simulink model "InductionCookerStateFlow_HarnessInductionCookerS11"  (R2023a)
settings: Solver=FixedStepDiscrete  StartTime=0.0  StopTime=2000  FixedStep=0.1  RelTol=1e-3  EnableMultiTasking=on
settings Model: Creator=antonio  LastModifiedBy=anton
settings SolverCC: AlgebraicLoopSolver=TrustRegion  AutoInsertRateTranBlk=on
settings DataIOCC: LimitDataPoints=on
settings OptimizationCC: LifeSpan=inf
settings DebuggingCC: UnconnectedInputMsg=warning  UnconnectedOutputMsg=warning  UnconnectedLineMsg=warning  AllowSymbolicDim=off  SFUnexpectedBacktrackingDiag=warning  SFNoUnconditionalDefaultTransitionDiag=warning  SFExecutionAtInitializationDiag=none  ArithmeticOperatorsInVariantConditions=warning
settings ModelReferenceCC: EnableRefExpFcnMdlSchedulingChecks=on
settings SFSimCC: SimUseLocalCustomCode=off  CustomCodeUndefinedFunction=UseInterfaceOnly
settings RTWCC: RTWUseLocalCustomCode=off  DLArmComputeVersion=19.05
settings CodeAppCC: StateflowObjectComments=on
settings GRTTargetCC: TargetLangStandard=C89/C90 (ANSI)
settings ConfigComp: CovEnable=on  RecordCoverage=on  CovMetricSettings=dw  CovSaveCumulativeToWorkspaceVar=on  CovSaveSingleToWorkspaceVar=on  CovModelRefEnable=on

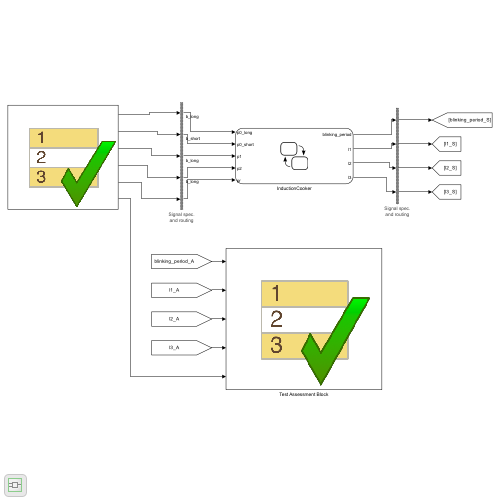
[thumbnail: Simulink's stored preview of the top-level diagram]
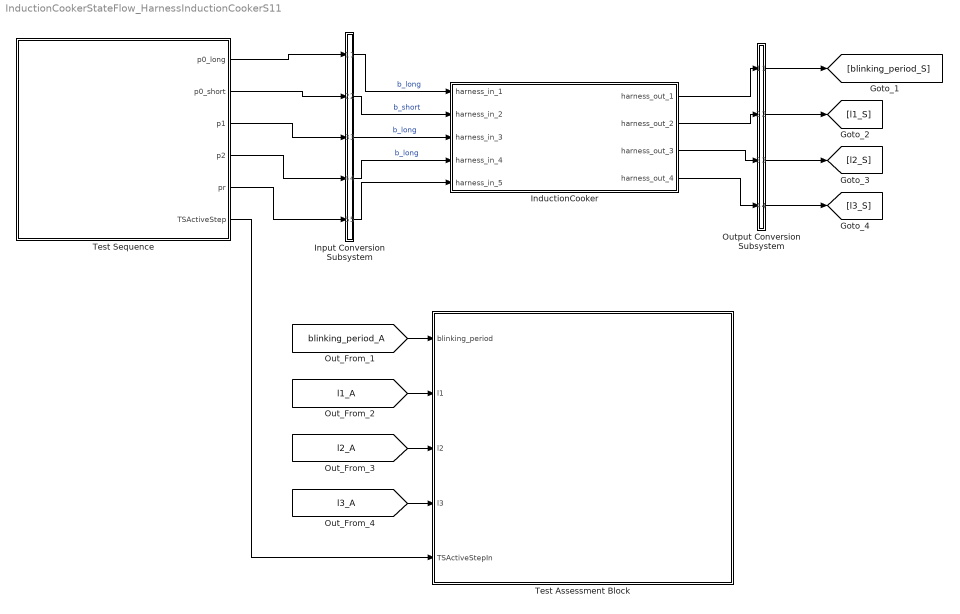
== system InductionCookerStateFlow_HarnessInductionCookerS11 ==
  InductionCooker : Subsystem  Tag=__SL_testing_harness_stub_
  Input Conversion Subsystem : Subsystem  Tag=__SLT_ICS__  Description=|
      | Signal spec.
      | and routing
      settings: AttributesFormatString=%<Description>
  Output Conversion Subsystem : Subsystem  Tag=__SLT_OCS__  Description=|
      | Signal spec.
      | and routing
      settings: AttributesFormatString=%<Description>
  Test Assessment Block : Test Sequence  Tag=__SLT_ASMT__  TreatAsAtomicUnit=on
  Test Sequence : Test Sequence  TreatAsAtomicUnit=on
  wires:
  [blinking_period_A] -> Test Assessment Block/1(blinking_period)
  [l1_A] -> Test Assessment Block/2(l1)
  [l2_A] -> Test Assessment Block/3(l2)
  [l3_A] -> Test Assessment Block/4(l3)
  Test Sequence/1(p0_long) -> Input Conversion Subsystem/1(Inport_1)
  Test Sequence/2(p0_short) -> Input Conversion Subsystem/2(Inport_2)
  Test Sequence/3(p1) -> Input Conversion Subsystem/3(Inport_3)
  Test Sequence/4(p2) -> Input Conversion Subsystem/4(Inport_4)
  Test Sequence/5(pr) -> Input Conversion Subsystem/5(Inport_5)
  Output Conversion Subsystem/1(Outport_1) -> [blinking_period_S]
  Output Conversion Subsystem/2(Outport_2) -> [l1_S]
  Output Conversion Subsystem/3(Outport_3) -> [l2_S]
  Output Conversion Subsystem/4(Outport_4) -> [l3_S]
  Test Sequence/6(TSActiveStep) -> Test Assessment Block/5(TSActiveStepIn)
  InductionCooker/1(harness_out_1) -> Output Conversion Subsystem/1(Inport_1)
  InductionCooker/2(harness_out_2) -> Output Conversion Subsystem/2(Inport_2)
  InductionCooker/3(harness_out_3) -> Output Conversion Subsystem/3(Inport_3)
  InductionCooker/4(harness_out_4) -> Output Conversion Subsystem/4(Inport_4)
  Input Conversion Subsystem/1(Outport_1) -> InductionCooker/1(harness_in_1)  "b_long"
  Input Conversion Subsystem/2(Outport_2) -> InductionCooker/2(harness_in_2)  "b_short"
  Input Conversion Subsystem/3(Outport_3) -> InductionCooker/3(harness_in_3)  "b_long"
  Input Conversion Subsystem/4(Outport_4) -> InductionCooker/4(harness_in_4)  "b_long"
  Input Conversion Subsystem/5(Outport_5) -> InductionCooker/5(harness_in_5)

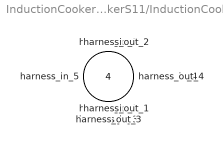
== system InductionCookerStateFlow_HarnessInductionCookerS11/InductionCooker ==
  harness_in_1 : Inport
  harness_in_2 : Inport  Port=2
  harness_in_3 : Inport  Port=3
  harness_in_4 : Inport  Port=4
  harness_in_5 : Inport  Port=5
  harness_out_1 : Outport
  harness_out_2 : Outport  Port=2
  harness_out_3 : Outport  Port=3
  harness_out_4 : Outport  Port=4

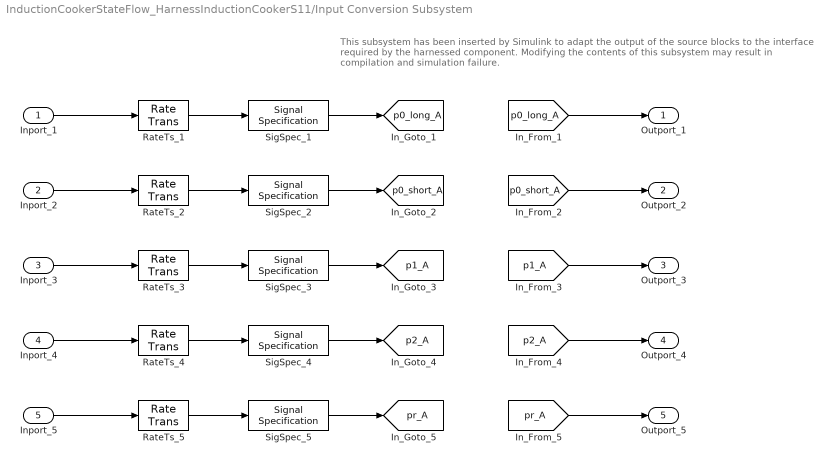
== system InductionCookerStateFlow_HarnessInductionCookerS11/Input Conversion Subsystem ==
  note: This subsystem has been inserted by Simulink to adapt the output of the source blocks to the interface required by the harnessed component.
      |  Modifying the contents of this subsystem may result in compilation and simulation failure.
  Inport_1 : Inport
  Inport_2 : Inport  Port=2
  Inport_3 : Inport  Port=3
  Inport_4 : Inport  Port=4
  Inport_5 : Inport  Port=5
  RateTs_{1..5} (5 alike) : RateTransition  OutPortSampleTime=0.1
  SigSpec_{1..5} (5 alike) : SignalSpecification  OutDataTypeStr=boolean  Dimensions=[1]  SampleTime=0.1
  Outport_1 : Outport
  Outport_2 : Outport  Port=2
  Outport_3 : Outport  Port=3
  Outport_4 : Outport  Port=4
  Outport_5 : Outport  Port=5
  tag scope: p0_long_A=global, p0_short_A=global, p1_A=global, p2_A=global, pr_A=global
  wires:
  [p0_long_A] -> Outport_1/1
  SigSpec_1/1 -> [p0_long_A]
  RateTs_1/1 -> SigSpec_1/1
  Inport_1/1 -> RateTs_1/1
  [p0_short_A] -> Outport_2/1
  SigSpec_2/1 -> [p0_short_A]
  RateTs_2/1 -> SigSpec_2/1
  Inport_2/1 -> RateTs_2/1
  [p1_A] -> Outport_3/1
  SigSpec_3/1 -> [p1_A]
  RateTs_3/1 -> SigSpec_3/1
  Inport_3/1 -> RateTs_3/1
  [p2_A] -> Outport_4/1
  SigSpec_4/1 -> [p2_A]
  RateTs_4/1 -> SigSpec_4/1
  Inport_4/1 -> RateTs_4/1
  [pr_A] -> Outport_5/1
  SigSpec_5/1 -> [pr_A]
  RateTs_5/1 -> SigSpec_5/1
  Inport_5/1 -> RateTs_5/1

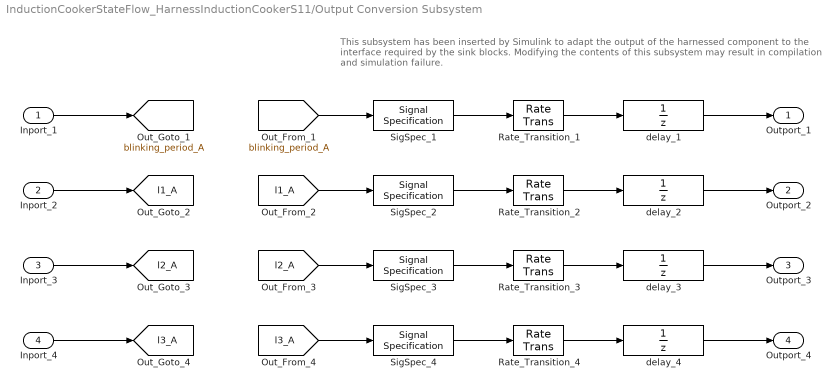
== system InductionCookerStateFlow_HarnessInductionCookerS11/Output Conversion Subsystem ==
  note: This subsystem has been inserted by Simulink to adapt the output of the harnessed component to the interface required by the sink blocks.
      |  Modifying the contents of this subsystem may result in compilation and simulation failure.
  Inport_1 : Inport
  Inport_2 : Inport  Port=2
  Inport_3 : Inport  Port=3
  Inport_4 : Inport  Port=4
  Rate_Transition_{1..4} (4 alike) : RateTransition  OutPortSampleTimeOpt=Inherit
  SigSpec_1 : SignalSpecification  OutDataTypeStr=uint32  Dimensions=[1]  SampleTime=0.1
  SigSpec_2 : SignalSpecification  OutDataTypeStr=boolean  Dimensions=[1]  SampleTime=0.1
  SigSpec_3 : SignalSpecification  OutDataTypeStr=boolean  Dimensions=[1]  SampleTime=0.1
  SigSpec_4 : SignalSpecification  OutDataTypeStr=boolean  Dimensions=[1]  SampleTime=0.1
  delay_{1..4} (4 alike) : UnitDelay  SampleTime=-1
  Outport_1 : Outport
  Outport_2 : Outport  Port=2
  Outport_3 : Outport  Port=3
  Outport_4 : Outport  Port=4
  tag scope: blinking_period_A=global, l1_A=global, l2_A=global, l3_A=global
  wires:
  Inport_1/1 -> [blinking_period_A]
  [blinking_period_A] -> SigSpec_1/1
  SigSpec_1/1 -> Rate_Transition_1/1
  Rate_Transition_1/1 -> delay_1/1
  delay_1/1 -> Outport_1/1
  Inport_2/1 -> [l1_A]
  [l1_A] -> SigSpec_2/1
  SigSpec_2/1 -> Rate_Transition_2/1
  Rate_Transition_2/1 -> delay_2/1
  delay_2/1 -> Outport_2/1
  Inport_3/1 -> [l2_A]
  [l2_A] -> SigSpec_3/1
  SigSpec_3/1 -> Rate_Transition_3/1
  Rate_Transition_3/1 -> delay_3/1
  delay_3/1 -> Outport_3/1
  Inport_4/1 -> [l3_A]
  [l3_A] -> SigSpec_4/1
  SigSpec_4/1 -> Rate_Transition_4/1
  Rate_Transition_4/1 -> delay_4/1
  delay_4/1 -> Outport_4/1

== stateflow chart InductionCookerStateFlow_HarnessInductionCookerS11/Test Assessment Block ==
  state Scenario_1
    state Run
      state VerifyInitS11
        verify(blinking_period == 0 & ~l1 & ~l2 & ~l3)
      state VerifyOnWithPotPresentS11
        verify(blinking_period == 0 & l1 & ~l2 & ~l3)
      state VerifyInactiveWithPotPresentS11
        verify(blinking_period == 0 & l1 & ~l2 & ~l3)
      state VerifyPowerIncreaseWithPotPresentS11
        verify(blinking_period == 0 & l1 & ~l2 & ~l3)
      state VerifyActive300WS11
        verify(blinking_period == 2000 & l1 & l2 & ~l3)
      state VerifyPowerIncreaseWithPotPresentAgainS11
        verify(blinking_period == 2000 & l1 & l2 & ~l3)
      state VerifyActive500WS11
        verify(blinking_period == 1000 & l1 & l2 & ~l3)
      state VerifyPowerIncreaseWithPotPresentAgain2S11
        verify(blinking_period == 1000 & l1 & l2 & ~l3)
      state VerifyActive100WS11
        verify(blinking_period == 500 & l1 & l2 & ~l3)
      state VerifyPowerIncreaseWithPotPresentAgain3S11
        verify(blinking_period == 500 & l1 & l2 & ~l3)
      state VerifyLongPressOffWithPotPresentS11
        verify(blinking_period == 0 & ~l1 & ~l2 & ~l3)
      state VerifyReleaseOffS11
        verify(blinking_period == 0 & ~l1 & ~l2 & ~l3)
      state step_1_2
      (default) -> (junction 1680)
      Run -> (junction 1680)
      (junction 1680) -> (junction 1681) [order 1] : [TSActiveStepIn == TSActiveStepEnumHInductionCooker.InitS11
          | ]
      (junction 1681) -> VerifyInitS11 [order 1] : [~in(Scenario_1.Run.VerifyInitS11)]
      (junction 1680) -> (junction 1690) [order 2]
      (junction 1681) -> (junction 1684) [order 2]
      (junction 1690) -> (junction 1691) [order 1] : [TSActiveStepIn == TSActiveStepEnumHInductionCooker.OnWithPotPresentS11
          | ]
      (junction 1691) -> VerifyOnWithPotPresentS11 [order 1] : [~in(Scenario_1.Run.VerifyOnWithPotPresentS11)]
      (junction 1690) -> (junction 1698) [order 2]
      (junction 1691) -> (junction 1694) [order 2]
      (junction 1698) -> (junction 1699) [order 1] : [TSActiveStepIn == TSActiveStepEnumHInductionCooker.InactiveWithPotPresentS11
          | ]
      (junction 1699) -> VerifyInactiveWithPotPresentS11 [order 1] : [~in(Scenario_1.Run.VerifyInactiveWithPotPresentS11)]
      (junction 1698) -> (junction 1706) [order 2]
      (junction 1699) -> (junction 1702) [order 2]
      (junction 1706) -> (junction 1707) [order 1] : [TSActiveStepIn == TSActiveStepEnumHInductionCooker.PowerIncreaseWithPotPresentS11
          | ]
      (junction 1707) -> VerifyPowerIncreaseWithPotPresentS11 [order 1] : [~in(Scenario_1.Run.VerifyPowerIncreaseWithPotPresentS11)]
      (junction 1706) -> (junction 1714) [order 2]
      (junction 1707) -> (junction 1710) [order 2]
      (junction 1714) -> (junction 1715) [order 1] : [TSActiveStepIn == TSActiveStepEnumHInductionCooker.Active300WS11
          | ]
      (junction 1715) -> VerifyActive300WS11 [order 1] : [~in(Scenario_1.Run.VerifyActive300WS11)]
      (junction 1714) -> (junction 1722) [order 2]
      (junction 1715) -> (junction 1718) [order 2]
      (junction 1722) -> (junction 1723) [order 1] : [TSActiveStepIn == TSActiveStepEnumHInductionCooker.PowerIncreaseWithPotPresentAgainS11
          | ]
      (junction 1723) -> VerifyPowerIncreaseWithPotPresentAgainS11 [order 1] : [~in(Scenario_1.Run.VerifyPowerIncreaseWithPotPresentAgainS11)]
      (junction 1722) -> (junction 1730) [order 2]
      (junction 1723) -> (junction 1726) [order 2]
      (junction 1730) -> (junction 1731) [order 1] : [TSActiveStepIn == TSActiveStepEnumHInductionCooker.Active500WS11
          | ]
      (junction 1731) -> VerifyActive500WS11 [order 1] : [~in(Scenario_1.Run.VerifyActive500WS11)]
      (junction 1730) -> (junction 1738) [order 2]
      (junction 1731) -> (junction 1734) [order 2]
      (junction 1738) -> (junction 1739) [order 1] : [TSActiveStepIn == TSActiveStepEnumHInductionCooker.PowerIncreaseWithPotPresentAgain2S11
          | ]
      (junction 1739) -> VerifyPowerIncreaseWithPotPresentAgain2S11 [order 1] : [~in(Scenario_1.Run.VerifyPowerIncreaseWithPotPresentAgain2S11)]
      (junction 1738) -> (junction 1773) [order 2]
      (junction 1739) -> (junction 1742) [order 2]
      (junction 1773) -> (junction 1774) [order 1] : [TSActiveStepIn == TSActiveStepEnumHInductionCooker.Active1000WS11
          | ]
      (junction 1774) -> VerifyActive100WS11 [order 1] : [~in(Scenario_1.Run.VerifyActive100WS11)]
      (junction 1782) -> (junction 1746) [order 2]
      (junction 1774) -> (junction 1777) [order 2]
      (junction 1782) -> (junction 1783) [order 1] : [TSActiveStepIn == TSActiveStepEnumHInductionCooker.PowerIncreaseWithPotPresentAgain3S11
          | ]
      (junction 1783) -> VerifyPowerIncreaseWithPotPresentAgain3S11 [order 1] : [~in(Scenario_1.Run.VerifyPowerIncreaseWithPotPresentAgain3S11)]
      (junction 1746) -> (junction 1747) [order 1] : [TSActiveStepIn == TSActiveStepEnumHInductionCooker.LongPressOffWithPotPresentS11
          | ]
      (junction 1747) -> VerifyLongPressOffWithPotPresentS11 [order 1] : [~in(Scenario_1.Run.VerifyLongPressOffWithPotPresentS11)]
      (junction 1746) -> (junction 1754) [order 2]
      (junction 1747) -> (junction 1750) [order 2]
      (junction 1754) -> (junction 1755) [order 1] : [TSActiveStepIn == TSActiveStepEnumHInductionCooker.ReleaseOffS11
          | ]
      (junction 1755) -> VerifyReleaseOffS11 [order 1] : [~in(Scenario_1.Run.VerifyReleaseOffS11)]
      (junction 1754) -> (junction 1762) [order 2]
      (junction 1755) -> (junction 1758) [order 2]
      (junction 1762) -> (junction 1763)
      (junction 1763) -> step_1_2 [order 1] : [~in(Scenario_1.Run.step_1_2)]
      (junction 1763) -> (junction 1766) [order 2]
      (junction 1783) -> (junction 1786) [order 2]
      (junction 1773) -> (junction 1782) [order 2]
    (default) -> Run
  (default) -> Scenario_1 : {assert(Active_Scenario_Index == 1,'The value of Scenario Parameter ''Active_Scenario_Index'' is not valid. Use the index of the scenario to specify it.')}
  data: blinking_period input uint32 size=[1]; l1 input boolean size=[1]; l2 input boolean size=[1]; l3 input boolean size=[1]; TSActiveStepIn input; Active_Scenario_Index parameter =1

== stateflow chart InductionCookerStateFlow_HarnessInductionCookerS11/Test Sequence ==
  settings: updateMethod=DISCRETE  sampleTime=0.1
  state Scenario_1
    state InitS11
      p0_long = true;
      p0_short = true;
      p1 = true;
      p2 = true;
      pr = false;
      settings: description=|
          | Condizione in cui tutti i pulsanti sono rilasciati e
          | la pentola è presente sul dispositivo.
    state OnWithPotPresentS11
      p0_long = true;
      p0_short = false;
      p1 = true;
      p2 = true;
      pr = false;
      settings: description=|
          | Condizione in cui il pulsante per l'accensione è
          | premuto, mentre tutti gli altri pulsanti sono
          | rilasciati e la pentola è presente sul dispositivo.
    state InactiveWithPotPresentS11
      p0_long = true;
      p0_short = true;
      p1 = true;
      p2 = true;
      pr = false;
      settings: description=|
          | Condizione in cui tutti i pulsanti sono rilasciati e la
          | pentola è presente sul dispositivo.
    state PowerIncreaseWithPotPresentS11
      p0_long = true;
      p0_short = true;
      p1 = false;
      p2 = true;
      pr =  false;
      settings: description=|
          | Condizione in cui il pulsante per l'aumento della
          | potenza è premuto per almeno 1 secondo, mentre
          | tutti gli altri pulsanti sono rilasciati e la pentola è
          | presente sul dispositivo.
    state Waiting300WS11
      p0_long = true;
      p0_short = true;
      p1 = true;
      p2 = true;
      pr =  false;
      settings: description=|
          | Condizione in cui tutti i pulsanti sono rilasciati
          | e la pentola è presente sul dispositivo.
          | Si attende che passino i 5 secondi per
          | l'effettivo cambio della potenza.
    state Active300WS11
      p0_long = true;
      p0_short = true;
      p1 = true;
      p2 = true;
      pr =  false;
      settings: description=|
          | Condizione in cui tutti i pulsanti sono rilasciati, la
          | pentola è presente sul dispositivo e quest'ultimo sta
          | erogando la potenza desiderata.
    state PowerIncreaseWithPotPresentAgainS11
      p0_long = true;
      p0_short = true;
      p1 = false;
      p2 = true;
      pr =  false;
      settings: description=|
          | Condizione in cui il pulsante per l'aumento della
          | potenza è premuto per almeno 1 secondo, mentre
          | tutti gli altri pulsanti sono rilasciati e la pentola è
          | presente sul dispositivo.
    state Waiting500WS11
      p0_long = true;
      p0_short = true;
      p1 = true;
      p2 = true;
      pr =  false;
      settings: description=|
          | Condizione in cui tutti i pulsanti sono rilasciati
          | e la pentola è presente sul dispositivo.
          | Si attende che passino i 5 secondi per
          | l'effettivo cambio della potenza.
    state Active500WS11
      p0_long = true;
      p0_short = true;
      p1 = true;
      p2 = true;
      pr =  false;
      settings: description=|
          | Condizione in cui tutti i pulsanti sono rilasciati, la
          | pentola è presente sul dispositivo e quest'ultimo sta
          | erogando la potenza desiderata.
    state PowerIncreaseWithPotPresentAgain2S11
      p0_long = true;
      p0_short = true;
      p1 = false;
      p2 = true;
      pr =  false;
      settings: description=|
          | Condizione in cui il pulsante per l'aumento della
          | potenza è premuto per almeno 1 secondo, mentre
          | tutti gli altri pulsanti sono rilasciati e la pentola è
          | presente sul dispositivo.
    state Waiting1000WS11
      p0_long = true;
      p0_short = true;
      p1 = true;
      p2 = true;
      pr =  false;
      settings: description=|
          | Condizione in cui tutti i pulsanti sono rilasciati
          | e la pentola è presente sul dispositivo.
          | Si attende che passino i 5 secondi per
          | l'effettivo cambio della potenza.
    state Active1000WS11
      p0_long = true;
      p0_short = true;
      p1 = true;
      p2 = true;
      pr =  false;
      settings: description=|
          | Condizione in cui tutti i pulsanti sono rilasciati, la
          | pentola è presente sul dispositivo e quest'ultimo sta
          | erogando la potenza desiderata.
    state PowerIncreaseWithPotPresentAgain3S11
      p0_long = true;
      p0_short = true;
      p1 = false;
      p2 = true;
      pr =  false;
      settings: description=|
          | Condizione in cui il pulsante per l'aumento della
          | potenza è premuto per almeno 1 secondo, mentre
          | tutti gli altri pulsanti sono rilasciati e la pentola è
          | presente sul dispositivo.
    state Waiting1500WS11
      p0_long = true;
      p0_short = true;
      p1 = true;
      p2 = true;
      pr =  false;
      settings: description=|
          | Condizione in cui tutti i pulsanti sono rilasciati
          | e la pentola è presente sul dispositivo.
          | Si attende che passino i 5 secondi per
          | l'effettivo cambio della potenza.
    state LongPressOffWithPotPresentS11
      p0_long = false;
      p0_short = true;
      p1 = true;
      p2 = true;
      pr =  false;
      settings: description=|
          | Condizione in cui il pulsante per lo spegnimento
          | è premuto per almeno 1 secondo, mentre tutti gli
          | altri pulsanti sono rilasciati e la pentola è presente
          | sul dispositivo.
    state ReleaseOffS11
      p0_long = true;
      p0_short = true;
      p1 = true;
      p2 = true;
      pr =  false;
      settings: description=|
          | Ritorno alla condizione iniziale rilasciando il
          | pulsante di spegnimento.
    (default) -> InitS11
    InitS11 -> OnWithPotPresentS11 : [
        | true
        | ]
    OnWithPotPresentS11 -> InactiveWithPotPresentS11 : [
        | true
        | ]
    InactiveWithPotPresentS11 -> PowerIncreaseWithPotPresentS11 : [
        | true
        | ]
    PowerIncreaseWithPotPresentS11 -> Waiting300WS11 : [
        | true
        | ]
    Waiting300WS11 -> Active300WS11 : [
        | after(5, sec)
        | ]
    Active300WS11 -> PowerIncreaseWithPotPresentAgainS11 : [
        | true
        | ]
    PowerIncreaseWithPotPresentAgainS11 -> Waiting500WS11 : [
        | true
        | ]
    Waiting500WS11 -> Active500WS11 : [
        | after(5, sec)
        | ]
    Active500WS11 -> PowerIncreaseWithPotPresentAgain2S11 : [
        | true
        | ]
    PowerIncreaseWithPotPresentAgain2S11 -> Waiting1000WS11 : [
        | true
        | ]
    Waiting1000WS11 -> Active1000WS11 : [
        | after(5,sec)
        | ]
    Active1000WS11 -> PowerIncreaseWithPotPresentAgain3S11 : [
        | true
        | ]
    PowerIncreaseWithPotPresentAgain3S11 -> Waiting1500WS11 : [
        | true
        | ]
    LongPressOffWithPotPresentS11 -> ReleaseOffS11 : [
        | true
        | ]
    Waiting1500WS11 -> LongPressOffWithPotPresentS11 : [
        | after(2,sec)
        | ]
  (default) -> Scenario_1 : {assert(Active_Scenario_Index == 1,'The value of Scenario Parameter ''Active_Scenario_Index'' is not valid. Use the index of the scenario to specify it.')}
  data: p0_long output boolean size=[1]; p0_short output boolean size=[1]; p1 output boolean size=[1]; p2 output boolean size=[1]; pr output boolean size=[1]; TSActiveStep output Enum: TSActiveStepEnumHInductionCooker; Active_Scenario_Index parameter =1
